simulink model "lab_exer_mat_4"  (R2015a)
settings: Solver=ode45  StartTime=0.0  StopTime=10.0  RelTol=1e-3
values from neighbouring files (symbols this model uses):
  Ts = 1    [Init_mat_4.m]
settings Model: Creator=nick  LastModifiedBy=nick

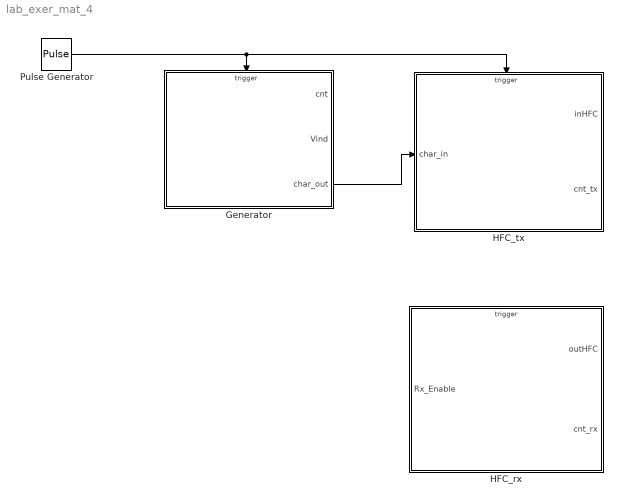
== system lab_exer_mat_4 ==
  Generator : Stateflow chart  TreatAsAtomicUnit=on
  HFC_rx : Stateflow chart  TreatAsAtomicUnit=on
  HFC_tx : Stateflow chart  TreatAsAtomicUnit=on
  Pulse Generator : DiscretePulseGenerator  PulseType=Time based  Period=Ts  PulseWidth=50
  wires:
  Pulse Generator/1 -> HFC_tx/Trigger, Generator/Trigger
  Generator/3(char_out) -> HFC_tx/1(char_in)

== stateflow chart lab_exer_mat_4/Generator ==
  state C [parallel]
    settings: executionOrder=1
    state UpCounter
      entry: upc = upc + 1;
      during: upc = upc + 1;
      UpCounter -> UpCounter
    (default) -> UpCounter : {upc=0;}
  state D [parallel]
    settings: executionOrder=2
    state S0
      entry: cnt = cnt + 1;
      ml.char_vals[cnt] = ml.randi(ml.Range, 1, 1);
      ml.fwrite(ml.s_port, ml.char_vals[cnt], 'uchar');
      ml.time_vals[cnt] = upc;
    state S_end
      entry: Vind = 1;
    state S1
    state S4
    state S3
    state S5
    state S2
    (default) -> S0 : {cnt=0;Vind=0;}
    S0 -> S_end [order 1] : [cnt==ml.Nc]
    (junction 70) -> S0
    S0 -> S1 [order 2]
    S3 -> S4
    S1 -> (junction 28) : {val=ml.rand(1);}
    S4 -> (junction 61) : {val=ml.rand(1);}
    S5 -> (junction 70)
    (junction 61) -> S5 [order 1] : [val>ml.qs[3]]
    (junction 34) -> S3 [order 1] : [val>ml.qs[2]]
    (junction 28) -> S2 [order 2] : [val>ml.qs[1]]
    S2 -> (junction 34) : {val=ml.rand(1);}
    (junction 34) -> (junction 70) [order 2] : [val<=ml.qs[2]]
    (junction 28) -> (junction 70) [order 1] : [val<=ml.qs[1]]
    (junction 61) -> (junction 70) [order 2] : [val<=ml.qs[3]]
  data: val local double; cnt output double; Vind output boolean; upc local int32; char_out output uint8
  events: clk input RISING_EDGE_EVENT

== stateflow chart lab_exer_mat_4/HFC_rx ==
  state Rx [parallel]
    settings: executionOrder=2
    state IniState
    state RxState
      en: ml('DIn_2');
      Val_rx = ml.d2r_s2;
      cnt_rx = cnt_rx + 1;
      ml.Rx_array[cnt_rx] = Val_rx;
    (default) -> IniState : {cnt_rx = 0;}
    (junction 174) -> IniState [order 1] : [ml.b2r_s2 == 0 ]
    IniState -> (junction 174) : {ml('B2R_2'); }
    (junction 174) -> RxState [order 2]
    RxState -> IniState
  state HFC_states [parallel]
    settings: executionOrder=1
    state HFCcon
      LBstatus_rx = Rx_Enable;
      ml.rts_s2 = LBstatus_rx;
      outHFC = LBstatus_rx;
      ml('RTS_2');
    state S2
    state S1
      LBstatus_rx = Rx_Enable;
    (default) -> HFCcon
    S2 -> HFCcon
    (junction 193) -> HFCcon [order 2]
    HFCcon -> (junction 193)
    (junction 202) -> HFCcon [order 2]
    (junction 193) -> S1 [order 1] : [LBstatus_rx == 0]
    (junction 202) -> S2 [order 1] : [LBstatus_rx == 0]
    S1 -> (junction 202)
  data: outHFC output double; Val_rx local uint8; cnt_rx output double; LBstatus_rx local double =0; Rx_Enable input
  events: clk input RISING_EDGE_EVENT

== stateflow chart lab_exer_mat_4/HFC_tx ==
  state IniState
    ml('CTS_1');
    LBstatus_tx = ml.cts_s1;
    inHFC = LBstatus_tx;
  state Dcalc
    en: ml('CTS_1');
    LBstatus_tx = ml.cts_s1;
    inHFC = LBstatus_tx;
  state Idle
  state TxState
    en: cnt_tx = cnt_tx + 1;
    ml.d2o_s1 = char_in;
    ml('DOut_1');
  (default) -> IniState : {cnt_tx = 0;}
  (junction 174) -> IniState [order 1] : [ml.b2o_s1 > 0 || LBstatus_tx == 0]
  IniState -> (junction 174) : {ml('B2O_1'); }
  (junction 174) -> Dcalc [order 2]
  (junction 194) -> IniState [order 2]
  Dcalc -> (junction 188)
  (junction 188) -> Dcalc [order 2]
  (junction 194) -> Idle [order 1] : [cnt_tx == ml.Ns]
  (junction 188) -> TxState [order 1] : [LBstatus_tx  ~= 0 ]
  TxState -> (junction 194)
  data: inHFC output double; cnt_tx output double; Val_tx local uint8; LBstatus_tx local double =0; char_in input uint8
  events: clk input RISING_EDGE_EVENT
